simulink model "IM_SpeedController_Design_ivdqsat"  (R2024b)
settings: Solver=VariableStepAuto  StartTime=0.0  StopTime=1+t_wstep  RelTol=1e-3
undefined symbols (not defined in the file): ctrl, en, im, J, lambda_Rd_ref, Lm, Lr, p, t_wstep, vSmax, w_amp
libraries: cstblocks x5, simulink x4
settings Model: Creator=overflow  LastModifiedBy=matth

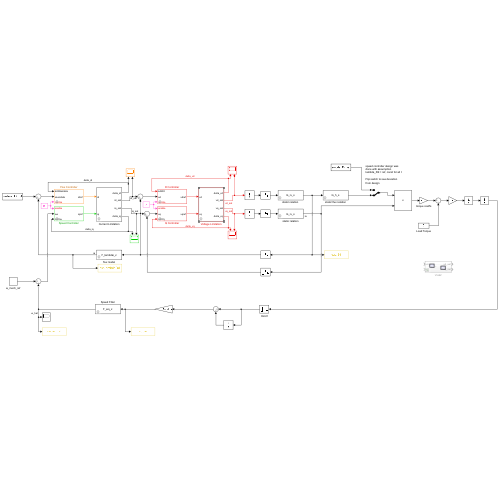
[thumbnail: Simulink's stored preview of the top-level diagram]
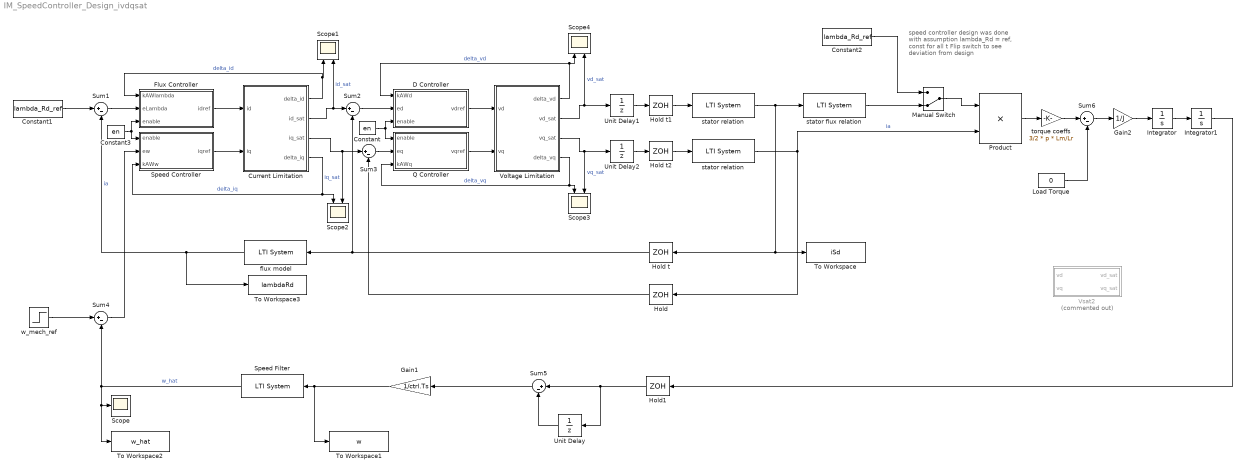
== system IM_SpeedController_Design_ivdqsat ==
  note: speed controller design was done with assumption lambda_Rd = ref, const for all t
      |
      | Flip switch to see deviation
      | from design
  " Hold" : ZeroOrderHold  SampleTime=ctrl.Ts
  " Hold t" : ZeroOrderHold  SampleTime=ctrl.Ts
  " Hold t1" : ZeroOrderHold  SampleTime=ctrl.Ts
  " Hold t2" : ZeroOrderHold  SampleTime=ctrl.Ts
  " Hold1" : ZeroOrderHold  SampleTime=ctrl.Ts
  Constant : Constant  Value=en
  Constant1 : Constant  Value=lambda_Rd_ref
  Constant2 : Constant  Value=lambda_Rd_ref
  Constant3 : Constant  Value=en
  Current Limitation : Subsystem  mask{Vmax=im.iSmax}
      mask prompts: Vmax "Max Voltage"
  D Controller : Subsystem  mask{Ts=ctrl.Ts, ctrl=ctrl.i}
      mask prompts: Ts "Sampling Time"; ctrl "Controller Struct"
  Flux Controller : Subsystem  mask{Ts=ctrl.Ts, ctrl=ctrl.lambdar}
      mask prompts: Ts "Sampling Time"; ctrl "Controller Struct"
  Gain1 : Gain  Gain=1/ctrl.Ts
  Gain2 : Gain  Gain=1/J
  Integrator : Integrator
  Integrator1 : Integrator
  Load Torque : Constant  Value=0
  Manual Switch : ManualSwitch  CurrentSetting=0
  Product : Product
  Q Controller : Subsystem  mask{Ts=ctrl.Ts, ctrl=ctrl.i}
      mask prompts: Ts "Sampling Time"; ctrl "Controller Struct"
  Scope : Scope
  Scope{1..4} (4 alike) : Scope  NumInputPorts=2
  Speed Controller : Subsystem  mask{Ts=ctrl.Ts, ctrl=ctrl.w}
      mask prompts: Ts "Sampling Time"; ctrl "Controller Struct"
  Speed Filter : cstblocks/LTI System  sys=F_wq_z  IC=[]  PadeOrder=0
      link override Internal: InitialCondition=w_start
  Sum{1..6} (6 alike) : Sum  Inputs=|+-
  To Workspace : ToWorkspace  VariableName=iSd  SaveFormat=Timeseries  SampleTime=-1
  To Workspace1 : ToWorkspace  VariableName=w  SaveFormat=Timeseries  SampleTime=-1
  To Workspace2 : ToWorkspace  VariableName=w_hat  SaveFormat=Timeseries  SampleTime=-1
  To Workspace3 : ToWorkspace  VariableName=lambdaRd  SaveFormat=Timeseries  SampleTime=-1
  Unit Delay : UnitDelay  SampleTime=-1  HasFrameUpgradeWarning=on
  Unit Delay1 : UnitDelay  SampleTime=ctrl.Ts  HasFrameUpgradeWarning=on
  Unit Delay2 : UnitDelay  SampleTime=ctrl.Ts  HasFrameUpgradeWarning=on
  Voltage Limitation : Subsystem  mask{Vmax=im.vSmax}
      mask prompts: Vmax "Max Voltage"
  Vsat2 : Subsystem  Commented=on
  flux model : cstblocks/LTI System  sys=F_lambdai_z  IC=[0]  PadeOrder=0
  stator flux relation : cstblocks/LTI System  sys=G_h_s  IC=[0]  PadeOrder=0
  stator relation : cstblocks/LTI System  sys=G_iv_s  IC=[0]  PadeOrder=0
  "stator relation " : cstblocks/LTI System  sys=G_iv_s  IC=[0]  PadeOrder=0
  torque coeffs : Gain  Gain=3/2 * p * Lm/Lr
  w_mech_ref : Step  Time=t_wstep  After=w_amp  SampleTime=0
  wires:
  Sum1/1 -> Flux Controller/2(eLambda)
  Sum2/1 -> D Controller/2(ed)
  Sum3/1 -> Q Controller/2(eq)
  Sum4/1 -> Speed Controller/2(ew)
  flux model/1 -> Sum1/2, To Workspace3/1  "ia"
  " Hold t"/1 -> Sum2/2, flux model/1
  " Hold t1"/1 -> "stator relation "/1
  " Hold t2"/1 -> stator relation/1
  " Hold"/1 -> Sum3/2
  "stator relation "/1 -> To Workspace/1, " Hold t"/1, stator flux relation/1
  stator relation/1 -> Product/2, " Hold"/1  "ia"
  Speed Filter/1 -> To Workspace2/1, Scope/1, Sum4/2  "w_hat"
  Unit Delay/1 -> Sum5/2
  " Hold1"/1 -> Unit Delay/1, Sum5/1
  Sum5/1 -> Gain1/1
  Integrator1/1 -> " Hold1"/1
  Load Torque/1 -> Sum6/2
  Product/1 -> torque coeffs/1
  torque coeffs/1 -> Sum6/1
  Sum6/1 -> Gain2/1
  Integrator/1 -> Integrator1/1
  Gain2/1 -> Integrator/1
  Gain1/1 -> To Workspace1/1, Speed Filter/1
  Unit Delay2/1 -> " Hold t2"/1
  Unit Delay1/1 -> " Hold t1"/1
  Constant1/1 -> Sum1/1
  w_mech_ref/1 -> Sum4/1
  stator flux relation/1 -> Manual Switch/2
  Manual Switch/1 -> Product/1
  Constant2/1 -> Manual Switch/1
  Voltage Limitation/3(vq_sat) -> Unit Delay2/1, Scope3/2  "vq_sat"
  Voltage Limitation/2(vd_sat) -> Scope4/2, Unit Delay1/1  "vd_sat"
  Q Controller/1(vqref) -> Voltage Limitation/2("vq ")
  D Controller/1(vdref) -> Voltage Limitation/1(vd)
  Constant/1 -> D Controller/3(enable), Q Controller/1(enable)
  Voltage Limitation/1(delta_vd) -> Scope4/1, D Controller/1(kAWd)  "delta_vd"
  Voltage Limitation/4(delta_vq) -> Scope3/1, Q Controller/3(kAWq)  "delta_vq"
  Current Limitation/3(iq_sat) -> Sum3/1, Scope2/2  "iq_sat"
  Current Limitation/2(id_sat) -> Sum2/1, Scope1/2  "id_sat"
  Current Limitation/4(delta_iq) -> Speed Controller/3(kAWw), Scope2/1  "delta_iq"
  Current Limitation/1(delta_id) -> Scope1/1, Flux Controller/1(kAWlambda)  "delta_id"
  Constant3/1 -> Speed Controller/1(enable), Flux Controller/3(enable)
  Flux Controller/1(idref) -> Current Limitation/1(id)
  Speed Controller/1(iqref) -> Current Limitation/2("iq ")

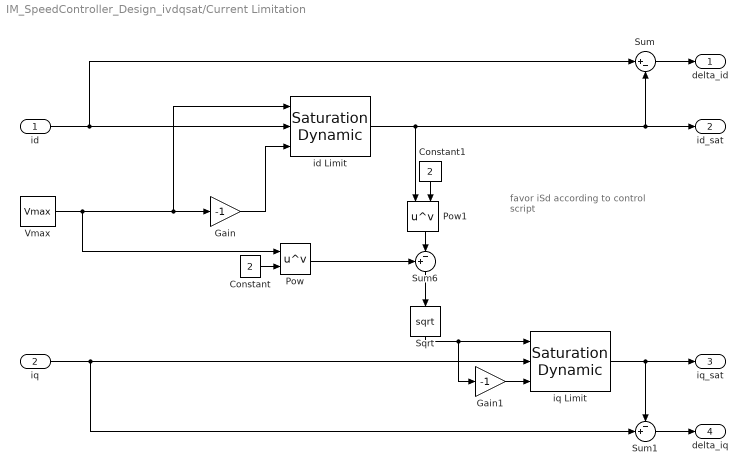
== system IM_SpeedController_Design_ivdqsat/Current Limitation ==
  note: favor iSd according
      | to control script
  id : Inport
  "iq " : Inport  Port=2
  Constant : Constant  Value=2
  Constant1 : Constant  Value=2
  Gain : Gain  Gain=-1
  Gain1 : Gain  Gain=-1
  Pow : Math  Operator=pow  RndMeth=Zero
  Pow1 : Math  Operator=pow  RndMeth=Zero
  Sqrt : Sqrt
  Sum : Sum  Inputs=|+-
  Sum1 : Sum  Inputs=-+|
  Sum6 : Sum  Inputs=+-|
  Vmax : Constant  Value=Vmax
  id Limit : simulink/Discontinuities/Saturation Dynamic  OutMin=[]  OutMax=[]  OutDataTypeStr=Inherit: Same as second input  OutDataType=fixdt(1, 16)  OutScaling=2^-10  DoSatur=off
  iq Limit : simulink/Discontinuities/Saturation Dynamic  OutMin=[]  OutMax=[]  OutDataTypeStr=Inherit: Same as second input  OutDataType=fixdt(1, 16)  OutScaling=2^-10  DoSatur=off
  delta_id : Outport  VectorParamsAs1DForOutWhenUnconnected=off
  id_sat : Outport  Port=2  VectorParamsAs1DForOutWhenUnconnected=off
  iq_sat : Outport  Port=3  VectorParamsAs1DForOutWhenUnconnected=off
  delta_iq : Outport  Port=4  VectorParamsAs1DForOutWhenUnconnected=off
  wires:
  Gain/1 -> id Limit/3
  id Limit/1 -> Sum/2, id_sat/1, Pow1/1
  Sqrt/1 -> Gain1/1, iq Limit/1
  iq Limit/1 -> Sum1/1, iq_sat/1
  Pow/1 -> Sum6/1
  id/1 -> Sum/1, id Limit/2
  Sum6/1 -> Sqrt/1
  "iq "/1 -> iq Limit/2, Sum1/2
  Pow1/1 -> Sum6/2
  Vmax/1 -> Pow/1, Gain/1, id Limit/1
  Gain1/1 -> iq Limit/3
  Sum/1 -> delta_id/1
  Sum1/1 -> delta_iq/1
  Constant/1 -> Pow/2
  Constant1/1 -> Pow1/2

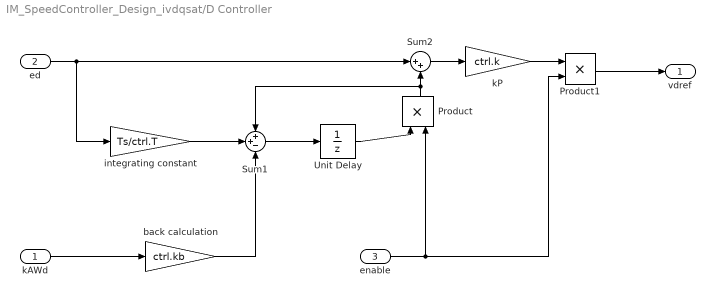
== system IM_SpeedController_Design_ivdqsat/D Controller ==
  kAWd : Inport
  ed : Inport  Port=2
  enable : Inport  Port=3
  Product : Product
  Product1 : Product
  Sum1 : Sum  Inputs=++-
  Sum2 : Sum  Inputs=|++
  Unit Delay : UnitDelay  SampleTime=-1  HasFrameUpgradeWarning=on
  back calculation : Gain  Gain=ctrl.kb
  integrating constant : Gain  Gain=Ts/ctrl.T
  kP : Gain  Gain=ctrl.k
  vdref : Outport
  wires:
  ed/1 -> integrating constant/1, Sum2/1
  Sum2/1 -> kP/1
  kAWd/1 -> back calculation/1
  Sum1/1 -> Unit Delay/1
  Unit Delay/1 -> Product/1
  Product/1 -> Sum1/1, Sum2/2
  kP/1 -> Product1/1
  Product1/1 -> vdref/1
  enable/1 -> Product1/2, Product/2
  integrating constant/1 -> Sum1/2
  back calculation/1 -> Sum1/3

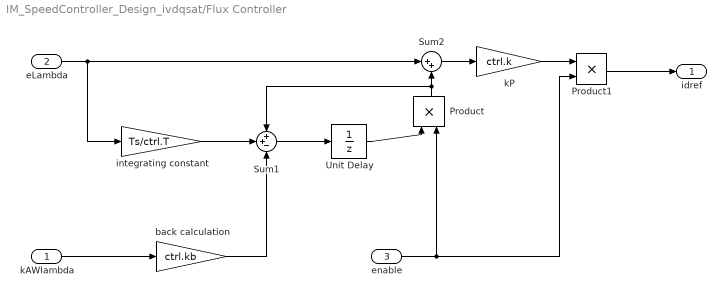
== system IM_SpeedController_Design_ivdqsat/Flux Controller ==
  kAWlambda : Inport
  eLambda : Inport  Port=2
  enable : Inport  Port=3
  Product : Product
  Product1 : Product
  Sum1 : Sum  Inputs=++-
  Sum2 : Sum  Inputs=|++
  Unit Delay : UnitDelay  SampleTime=-1  HasFrameUpgradeWarning=on
  back calculation : Gain  Gain=ctrl.kb
  integrating constant : Gain  Gain=Ts/ctrl.T
  kP : Gain  Gain=ctrl.k
  idref : Outport
  wires:
  eLambda/1 -> integrating constant/1, Sum2/1
  Sum2/1 -> kP/1
  kAWlambda/1 -> back calculation/1
  Sum1/1 -> Unit Delay/1
  Unit Delay/1 -> Product/1
  Product/1 -> Sum1/1, Sum2/2
  kP/1 -> Product1/1
  Product1/1 -> idref/1
  enable/1 -> Product1/2, Product/2
  integrating constant/1 -> Sum1/2
  back calculation/1 -> Sum1/3

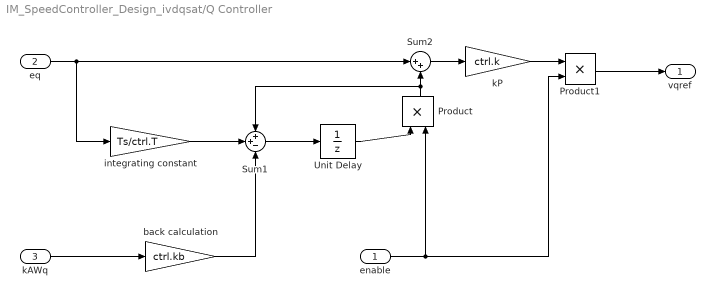
== system IM_SpeedController_Design_ivdqsat/Q Controller ==
  enable : Inport
  eq : Inport  Port=2
  kAWq : Inport  Port=3
  Product : Product
  Product1 : Product
  Sum1 : Sum  Inputs=++-
  Sum2 : Sum  Inputs=|++
  Unit Delay : UnitDelay  SampleTime=-1  HasFrameUpgradeWarning=on
  back calculation : Gain  Gain=ctrl.kb
  integrating constant : Gain  Gain=Ts/ctrl.T
  kP : Gain  Gain=ctrl.k
  vqref : Outport
  wires:
  eq/1 -> integrating constant/1, Sum2/1
  Sum2/1 -> kP/1
  kAWq/1 -> back calculation/1
  Sum1/1 -> Unit Delay/1
  Unit Delay/1 -> Product/1
  Product/1 -> Sum1/1, Sum2/2
  kP/1 -> Product1/1
  Product1/1 -> vqref/1
  enable/1 -> Product1/2, Product/2
  integrating constant/1 -> Sum1/2
  back calculation/1 -> Sum1/3

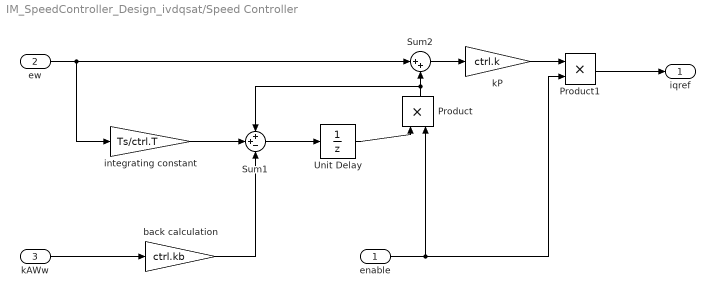
== system IM_SpeedController_Design_ivdqsat/Speed Controller ==
  enable : Inport
  ew : Inport  Port=2
  kAWw : Inport  Port=3
  Product : Product
  Product1 : Product
  Sum1 : Sum  Inputs=++-
  Sum2 : Sum  Inputs=|++
  Unit Delay : UnitDelay  SampleTime=-1  HasFrameUpgradeWarning=on
  back calculation : Gain  Gain=ctrl.kb
  integrating constant : Gain  Gain=Ts/ctrl.T
  kP : Gain  Gain=ctrl.k
  iqref : Outport
  wires:
  ew/1 -> integrating constant/1, Sum2/1
  Sum2/1 -> kP/1
  kAWw/1 -> back calculation/1
  Sum1/1 -> Unit Delay/1
  Unit Delay/1 -> Product/1
  Product/1 -> Sum1/1, Sum2/2
  kP/1 -> Product1/1
  Product1/1 -> iqref/1
  enable/1 -> Product1/2, Product/2
  integrating constant/1 -> Sum1/2
  back calculation/1 -> Sum1/3

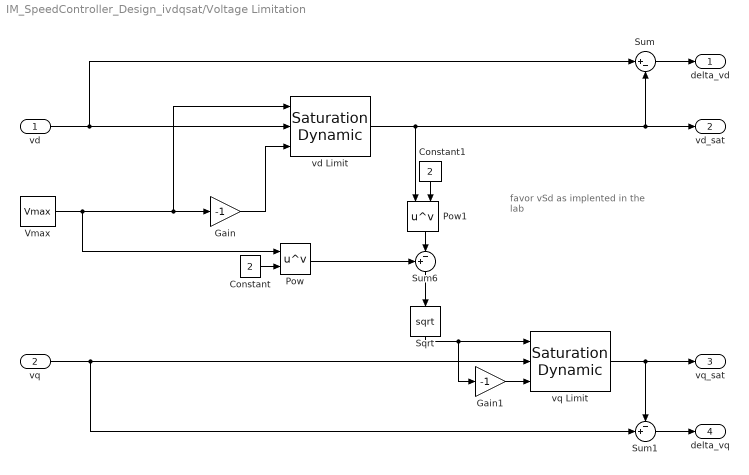
== system IM_SpeedController_Design_ivdqsat/Voltage Limitation ==
  note: favor vSd as implented in the lab
  vd : Inport
  "vq " : Inport  Port=2
  Constant : Constant  Value=2
  Constant1 : Constant  Value=2
  Gain : Gain  Gain=-1
  Gain1 : Gain  Gain=-1
  Pow : Math  Operator=pow  RndMeth=Zero
  Pow1 : Math  Operator=pow  RndMeth=Zero
  Sqrt : Sqrt
  Sum : Sum  Inputs=|+-
  Sum1 : Sum  Inputs=-+|
  Sum6 : Sum  Inputs=+-|
  Vmax : Constant  Value=Vmax
  vd Limit : simulink/Discontinuities/Saturation Dynamic  OutMin=[]  OutMax=[]  OutDataTypeStr=Inherit: Same as second input  OutDataType=fixdt(1, 16)  OutScaling=2^-10  DoSatur=off
  vq Limit : simulink/Discontinuities/Saturation Dynamic  OutMin=[]  OutMax=[]  OutDataTypeStr=Inherit: Same as second input  OutDataType=fixdt(1, 16)  OutScaling=2^-10  DoSatur=off
  delta_vd : Outport  VectorParamsAs1DForOutWhenUnconnected=off
  vd_sat : Outport  Port=2  VectorParamsAs1DForOutWhenUnconnected=off
  vq_sat : Outport  Port=3  VectorParamsAs1DForOutWhenUnconnected=off
  delta_vq : Outport  Port=4  VectorParamsAs1DForOutWhenUnconnected=off
  wires:
  Gain/1 -> vd Limit/3
  vd Limit/1 -> Sum/2, vd_sat/1, Pow1/1
  Sqrt/1 -> Gain1/1, vq Limit/1
  vq Limit/1 -> Sum1/1, vq_sat/1
  Pow/1 -> Sum6/1
  vd/1 -> Sum/1, vd Limit/2
  Sum6/1 -> Sqrt/1
  "vq "/1 -> vq Limit/2, Sum1/2
  Pow1/1 -> Sum6/2
  Vmax/1 -> Pow/1, Gain/1, vd Limit/1
  Gain1/1 -> vq Limit/3
  Sum/1 -> delta_vd/1
  Sum1/1 -> delta_vq/1
  Constant/1 -> Pow/2
  Constant1/1 -> Pow1/2

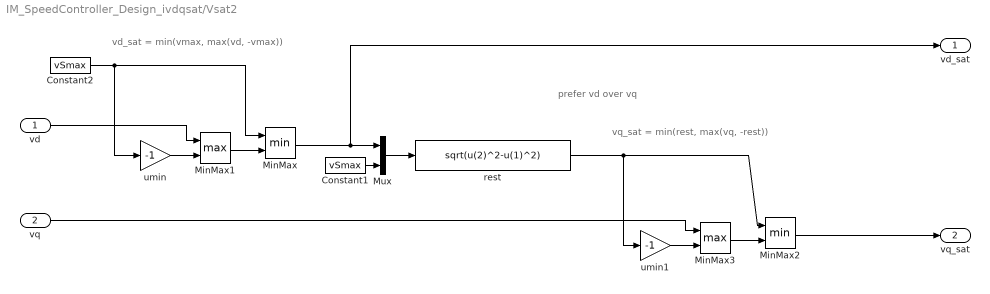
== system IM_SpeedController_Design_ivdqsat/Vsat2 ==
  note: prefer vd over vq
  note: vq_sat = min(rest, max(vq, -rest))
  note: vd_sat = min(vmax, max(vd, -vmax))
  vd : Inport
  vq : Inport  Port=2
  Constant1 : Constant  Value=vSmax
  Constant2 : Constant  Value=vSmax
  MinMax : MinMax  Inputs=2  InputSameDT=on  SaturateOnIntegerOverflow=on
  MinMax1 : MinMax  Function=max  Inputs=2  InputSameDT=on  SaturateOnIntegerOverflow=on
  MinMax2 : MinMax  Inputs=2  InputSameDT=on  SaturateOnIntegerOverflow=on
  MinMax3 : MinMax  Function=max  Inputs=2  InputSameDT=on  SaturateOnIntegerOverflow=on
  Mux : Mux  Inputs=2
  rest : Fcn  Expr=sqrt(u(2)^2-u(1)^2)
  umin : Gain  Gain=-1  SaturateOnIntegerOverflow=on  OutDataTypeStr=Inherit: Same as input  ParamDataTypeStr=Inherit: Same as input
  umin1 : Gain  Gain=-1  SaturateOnIntegerOverflow=on  OutDataTypeStr=Inherit: Same as input  ParamDataTypeStr=Inherit: Same as input
  vd_sat : Outport
  vq_sat : Outport  Port=2
  wires:
  MinMax/1 -> vd_sat/1, Mux/1
  Constant2/1 -> umin/1, MinMax/1
  MinMax1/1 -> MinMax/2
  umin/1 -> MinMax1/2
  vd/1 -> MinMax1/1
  Mux/1 -> rest/1
  Constant1/1 -> Mux/2
  umin1/1 -> MinMax3/2
  MinMax3/1 -> MinMax2/2
  rest/1 -> MinMax2/1, umin1/1
  MinMax2/1 -> vq_sat/1
  vq/1 -> MinMax3/1
